simulink model "cheat_sheat"  (R2018b)
settings: Solver=VariableStepAuto  StartTime=0.0  StopTime=10.0  RelTol=1e-3
settings Model: Creator=victo  LastModifiedBy=victo

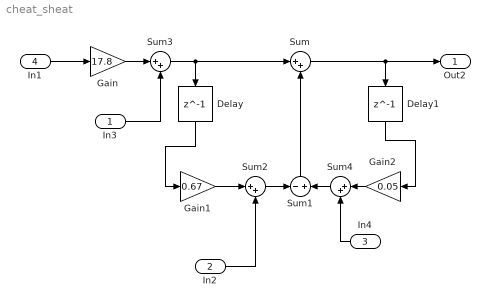
== system cheat_sheat ==
  In3 : Inport  OutMin=[-1]  OutMax=[1]
  In2 : Inport  Port=2  OutMin=[-1]  OutMax=[1]
  In4 : Inport  Port=3  OutMin=[-1]  OutMax=[1]
  In1 : Inport  Port=4  OutMin=[-1]  OutMax=[1]
  Delay : Delay  DelayLength=1
  Delay1 : Delay  DelayLength=1
  Gain : Gain  Gain=17.8
  Gain1 : Gain  Gain=0.67
  Gain2 : Gain  Gain=0.05
  Sum{,2..4} (4 alike) : Sum  Inputs=|++
  Sum1 : Sum  Inputs=-+
  Out2 : Outport
  wires:
  Delay1/1 -> Gain2/1
  Sum/1 -> Delay1/1, Out2/1
  Delay/1 -> Gain1/1
  Sum1/1 -> Sum/2
  In1/1 -> Gain/1
  Sum2/1 -> Sum1/1
  Gain1/1 -> Sum2/1
  In2/1 -> Sum2/2
  Gain/1 -> Sum3/1
  In3/1 -> Sum3/2
  Sum3/1 -> Sum/1, Delay/1
  Sum4/1 -> Sum1/2
  Gain2/1 -> Sum4/1
  In4/1 -> Sum4/2
